simulink model "Comau_endeff_Comp"  (R2024b)
settings: Solver=FixedStepAuto  StartTime=0.0  StopTime=inf  FixedStep=Ts  RelTol=1e-3
model workspace (MATLAB code in the model file):
  other statements: smiDataRobot.RigidTransform(16).translation = [0.0 0.0 0.0];; smiDataRobot.RigidTransform(16).angle = 0.0;; smiDataRobot.RigidTransform(16).axis = [0.0 0.0 0.0];; smiDataRobot.RigidTransform(16).ID = "";; smiDataRobot.RigidTransform(1).translation = [0 331 0];  % mm; smiDataRobot.RigidTransform(1).angle = 0;  % rad; smiDataRobot.RigidTransform(1).axis = [0 0 0];; smiDataRobot.RigidTransform(1).ID = "AssemblyGround[SMART-5 NJ-110-3.0 (3D-STEP).STEP-1:SMART-5 NJ-110-3.0_p02.STEP-1]";; smiDataRobot.RigidTransform(2).translation = [-450 2240 0];  % mm; smiDataRobot.RigidTransform(2).angle = 0;  % rad; smiDataRobot.RigidTransform(2).axis = [0 0 0];; smiDataRobot.RigidTransform(2).ID = "AssemblyGround[SMART-5 NJ-110-3.0 (3D-STEP).STEP-1:SMART-5 NJ-110-3.0_p05.STEP-1]"; ... (+161)
values from neighbouring files (symbols this model uses):
  BList = Adjoint(M_B) * SList    [Comau_robot_3dof_parameters.m]
  M = [1 0 0 L1+L5+L6+L7 ... (first row only)    [Comau_robot_3dof_parameters.m]
  M_B = TransInv(M)    [Comau_robot_3dof_parameters.m]
  SList = [omega_mat; v_mat]    [Comau_robot_3dof_parameters.m]
  thetaList0 = [0 0 0 0 0]    [Comau_robot_3dof_parameters.m]
  tr_p_c = [-1.082024099747949, 1.536041691521612, -0.3]    [Comau_robot_3dof_parameters.m]
  tr_w_p = [-2.969661622702265, 1.976311036084776, 3.312845015592614]    [Comau_robot_3dof_parameters.m]
undefined symbols (not defined in the file or in its folder): L2, L3, L4, SF_x, SF_y, SF_z, smiDataRobot, X, Y, Z
libraries: sm_lib x96, nesl_utility x69, slrealtimeutilitieslib x2, slrealtimeiplib x2, simulink x1, aerolibanimutils x1
(part 5 of 5)

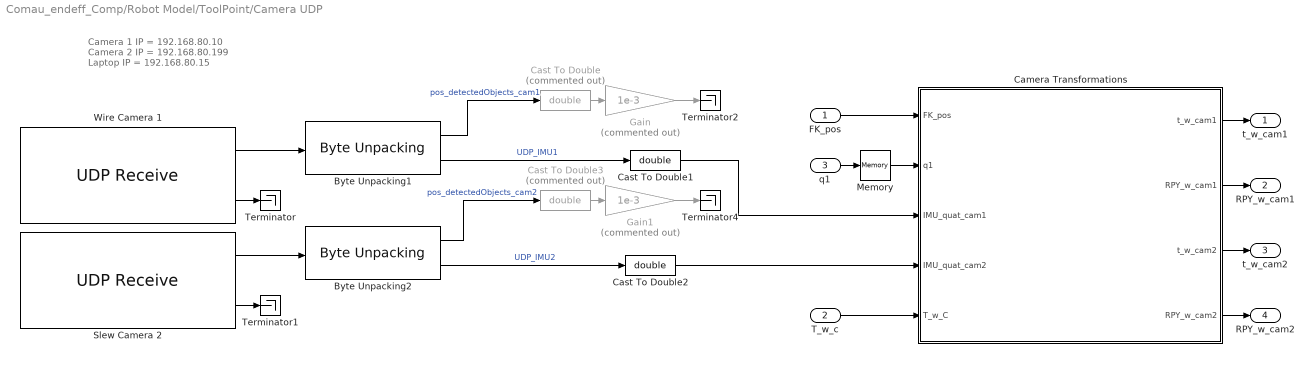
== system Comau_endeff_Comp/Robot Model/ToolPoint/Camera UDP ==
  note: Camera 1 IP = 192.168.80.10
      | Camera 2 IP = 192.168.80.199
      | Laptop IP      = 192.168.80.15
  FK_pos : Inport
  T_w_c : Inport  Port=2
  q1 : Inport  Port=3
  Byte Unpacking1 : slrealtimeutilitieslib/Byte Unpacking  MaskUnpackedDataTypes={'int16', 'single'}  MaskUnpackedDataSizes={[6], [4]}  MaskAlignment=1
  Byte Unpacking2 : slrealtimeutilitieslib/Byte Unpacking  MaskUnpackedDataTypes={'int16', 'single'}  MaskUnpackedDataSizes={[6], [4]}  MaskAlignment=1
  Camera Transformations : MATLAB Function  TreatAsAtomicUnit=on
  Cast To Double : DataTypeConversion  Commented=on  OutDataTypeStr=double  SaturateOnIntegerOverflow=off  RndMeth=Floor
  Cast To Double1 : DataTypeConversion  OutDataTypeStr=double  SaturateOnIntegerOverflow=off  RndMeth=Floor
  Cast To Double2 : DataTypeConversion  OutDataTypeStr=double  SaturateOnIntegerOverflow=off  RndMeth=Floor
  Cast To Double3 : DataTypeConversion  Commented=on  OutDataTypeStr=double  SaturateOnIntegerOverflow=off  RndMeth=Floor
  Gain : Gain  Commented=on  Gain=1e-3
  Gain1 : Gain  Commented=on  Gain=1e-3
  Memory : Memory
  Slew Camera 2 : slrealtimeiplib/UDP Receive  useHostTargetConn=on  ipAddress=192.168.5.80  localPort=5007  rcvWidth=28  rcvFmAny=on  fmAddress='10.10.10.10'  sampleTime=Ts  enableMessage=off  maxPackets=1
  Terminator{,1..2,4} (4 alike) : Terminator
  Wire Camera 1 : slrealtimeiplib/UDP Receive  useHostTargetConn=on  ipAddress=192.168.5.80  localPort=5008  rcvWidth=28  rcvFmAny=on  fmAddress='10.10.10.10'  sampleTime=Ts  enableMessage=off  maxPackets=1
  t_w_cam1 : Outport
  RPY_w_cam1 : Outport  Port=2
  t_w_cam2 : Outport  Port=3
  RPY_w_cam2 : Outport  Port=4
  wires:
  Byte Unpacking1/1 -> Cast To Double/1  "pos_detectedObjects_cam1"
  Wire Camera 1/1 -> Byte Unpacking1/1
  Wire Camera 1/2 -> Terminator/1
  Byte Unpacking1/2 -> Cast To Double1/1  "UDP_IMU1"
  Cast To Double/1 -> Gain/1
  FK_pos/1 -> Camera Transformations/1(FK_pos)
  Camera Transformations/1(t_w_cam1) -> t_w_cam1/1
  Cast To Double1/1 -> Camera Transformations/3(IMU_quat_cam1)
  Camera Transformations/2(RPY_w_cam1) -> RPY_w_cam1/1
  q1/1 -> Memory/1
  Memory/1 -> Camera Transformations/2(q1)
  T_w_c/1 -> Camera Transformations/5(T_w_C)
  Camera Transformations/4(RPY_w_cam2) -> RPY_w_cam2/1
  Camera Transformations/3(t_w_cam2) -> t_w_cam2/1
  Slew Camera 2/2 -> Terminator1/1
  Slew Camera 2/1 -> Byte Unpacking2/1
  Cast To Double2/1 -> Camera Transformations/4(IMU_quat_cam2)
  Byte Unpacking2/2 -> Cast To Double2/1  "UDP_IMU2"
  Byte Unpacking2/1 -> Cast To Double3/1  "pos_detectedObjects_cam2"
  Gain/1 -> Terminator2/1
  Cast To Double3/1 -> Gain1/1
  Gain1/1 -> Terminator4/1

== matlab function Comau_endeff_Comp/TrajectoryGen ==
  settings: updateMethod=DISCRETE
  data: points_x input; points_y input; points_z input; p output size=[1 3]; t input; t_points input; new_command input; traj_method input; p_vel output size=[1 3]; v_max input; traj_running output boolean size=1
function [p, p_vel, traj_running] = TrajectoryGen(points_x, points_y, points_z, t, t_points, new_command, traj_method, v_max)
%#codegen
% TrajectoryGen generates a 3D trajectory based on input waypoints.
%
% Inputs:
%   points_x, points_y, points_z - waypoint vectors or single values
%   depending on trajecotry generator mode (traj_method)
%   t      - current time (scalar)
%   t_points - vector of time stamps for the trajectory
%   new_command - a command counter (as single)
%
% Outputs:
%   p, p_vel - current position and velocity (1x3 vectors)
%   abs_tf_log, base_t_log, local_t, local_tf - diagnostic time variables

% Pre-allocate outputs:
p = zeros(1, 3);
p_vel = zeros(1, 3);

%Traj method for poly spline trajectory
%method = 'quintic';

% Persistent variables for timing and command tracking, and to hold new parameters:
persistent abs_tf base_t last_command 
persistent new_points_x new_points_y new_points_z new_t_points

% Removed cast: t = single(t);

if isempty(abs_tf)
    base_t = 0;
    abs_tf = 0;
end
if isempty(last_command)
    last_command = 0;
end

% Initialize captured parameters if empty:
if isempty(new_points_x)
    new_points_x = points_x;
end
if isempty(new_points_y)
    new_points_y = points_y;
end
if isempty(new_points_z)
    new_points_z = points_z;
end
if isempty(new_t_points)
    new_t_points = t_points;
end

% Detect a new trajectory command:
if new_command ~= last_command
    % Capture the current time as the start:
    base_t = t;
    
    % Capture the new parameters so they remain consistent:
    new_points_x = points_x;
    new_points_y = points_y;
    new_points_z = points_z;
    
    % Calculate the trajectory duration T based on Vmax.
    % Ensure Vmax is not too small and set a minimum time:
    T_min = 1e-6;
    v_max = max(v_max, T_min);
    
    % For a two-point trajectory, use the difference between the first two points.
    T_x = abs(new_points_x(2) - new_points_x(1)) / v_max;
    T_y = abs(new_points_y(2) - new_points_y(1)) / v_max;
    T_z = abs(new_points_z(2) - new_points_z(1)) / v_max;
    
    % Choose the maximum time required among all three axes:
    T = max([T_x, T_y, T_z, T_min]);
    
    % Set the absolute finish time based on the computed duration:
    abs_tf = T + t;
    
    % (Optionally) store T in new_t_points if needed
    new_t_points = T;  
    
    % Update the command counter:
    last_command = new_command;
end

% Compute local time variables:
local_t = t - base_t;
local_tf = abs_tf - base_t;


%maybe not need keep for now
% Clamp local_t so it doesn't exceed the final time:
%if traj_method ~= 3
%    if local_t > local_tf
%        local_t = local_tf;
%    end
%end

% Compute the trajectory:
if abs_tf == 0 || v_max == 0 % Stay in current position if Trajectory not initialized OR v_max input = 0
    x_pos = new_points_x(1);
    y_pos = new_points_y(1);
    z_pos = new_points_z(1);
    
    x_vel = 0;
    y_vel = 0;
    z_vel = 0;
else
    if traj_method == 1
        [x_pos, x_vel, ~] = cubicTrajectoryPlanner(local_t, local_tf, new_points_x(1), new_points_x(2), 0, 0);
        [y_pos, y_vel, ~] = cubicTrajectoryPlanner(local_t, local_tf, new_points_y(1), new_points_y(2), 0, 0);
        [z_pos, z_vel, ~] = cubicTrajectoryPlanner(local_t, local_tf, new_points_z(1), new_points_z(2), 0, 0);
        
        %VMax
        %[x_pos, x_vel, ~] = cubicTrajectoryPlanner_Vmax(local_t, v_max, new_points_x(1), new_points_x(2), 0, 0);
        %[y_pos, y_vel, ~] = cubicTrajectoryPlanner_Vmax(local_t, v_max, new_points_y(1), new_points_y(2), 0, 0);
        %[z_pos, z_vel, ~] = cubicTrajectoryPlanner_Vmax(local_t, v_max, new_points_z(1), new_points_z(2), 0, 0);
    elseif traj_method == 2
        %Quintic [pos, vel, acc] = quinticTrajectoryPlanner(t, T, P0, Pf, V0, Vf, A0, Af)
        [x_pos, x_vel, ~] = quinticTrajectoryPlanner(local_t, local_tf, new_points_x(1), new_points_x(2), 0, 0, 0, 0);
        [y_pos, y_vel, ~] = quinticTrajectoryPlanner(local_t, local_tf, new_points_y(1), new_points_y(2), 0, 0, 0, 0);
        [z_pos, z_vel, ~] = quinticTrajectoryPlanner(local_t, local_tf, new_points_z(1), new_points_z(2), 0, 0, 0, 0);
        
        %VMax
        %[x_pos, x_vel, ~] = quinticTrajectoryPlanner_Vmax(local_t, v_max, new_points_x(1), new_points_x(2), 0, 0, 0, 0);
        %[y_pos, y_vel, ~] = quinticTrajectoryPlanner_Vmax(local_t, v_max, new_points_y(1), new_points_y(2), 0, 0, 0, 0);
        %[z_pos, z_vel, ~] = quinticTrajectoryPlanner_Vmax(local_t, v_max, new_points_z(1), new_points_z(2), 0, 0, 0, 0);
    elseif traj_method == 3
        method = 'quintic';
        %Multi point online trajectory planner here
        %[x_pos, x_vel, ~, ~] = multipointTrajectorySplineAuto(local_t, new_points_x, v_max, method);
        %[y_pos, y_vel, ~, ~] = multipointTrajectorySplineAuto(local_t, new_points_y, v_max, method);
        %[z_pos, z_vel, ~, ~] = multipointTrajectorySplineAuto(local_t, new_points_z, v_max, method);

        x_pos = new_points_x(1);
        y_pos = new_points_y(1);
        z_pos = new_points_z(1);
        
        x_vel = 0;
        y_vel = 0;
        z_vel = 0;
    else %Defualt cubic
        [x_pos, x_vel, ~] = cubicTrajectoryPlanner(local_t, local_tf, new_points_x(1), new_points_x(2), 0, 0);
        [y_pos, y_vel, ~] = cubicTrajectoryPlanner(local_t, local_tf, new_points_y(1), new_points_y(2), 0, 0);
        [z_pos, z_vel, ~] = cubicTrajectoryPlanner(local_t, local_tf, new_points_z(1), new_points_z(2), 0, 0);
    end
end


p(1) = x_pos;
p(2) = y_pos;
p(3) = z_pos;

p_vel(1) = x_vel;
p_vel(2) = y_vel;
p_vel(3) = z_vel;

traj_running = (t <= abs_tf + 0.1); %Trajectory complete flag with 0.1 second buffer

traj_running = logical(traj_running);
end

== matlab function Comau_endeff_Comp/Robot Model/ToolPoint/Camera UDP/Camera Transformations ==
  data: t_w_cam1 output; FK_pos input; q1 input; IMU_quat_cam1 input; IMU_quat_cam2 input; RPY_w_cam1 output; t_w_cam2 output; T_w_C input; RPY_w_cam2 output
function [t_w_cam1, RPY_w_cam1, t_w_cam2, RPY_w_cam2] = transformFrame(FK_pos, q1, IMU_quat_cam1, IMU_quat_cam2, T_w_C)

    % FK_pos = t_w_ee
% World to End Effector
R_w_ee = rotz_deg(-q1);
% t_C_ee_homog = [FK_pos; 1];
% t_w_ee_homog = T_w_C * t_C_ee_homog;
% t_w_ee = t_w_ee_homog(1:3);
t_w_ee = FK_pos + T_w_C(1:3, 4);
T_w_ee = [R_w_ee, t_w_ee; 
           0 0 0,      1 ];

%%% Common for all OAK D Pro Cameras %%%
% Camera frame to IMU
R_cam_IMU = roty_deg(-90);
t_cam_IMU = [-1.18 ; 4.50 ; -27.25 ]*1e-3; % [m]
T_cam_IMU = [R_cam_IMU , t_cam_IMU;
                 0 0 0 ,         1 ];

% % Camera frame to RGB
% R_cam_RGB = 0; % <<<<<<<<<<<<<<<<<<<<<<<<<<<<<<<<<<<<<<<
% t_cam_RGB = [ 7.2 ; 44.5 ; -6.9867 ]*1e-3; % [m]
% T_cam_RGB = [ R_cam_RGB , t_cam_RGB;
%                   0 0 0 ,         1 ];
%%% Common for all OAK D Pro Cameras %%%

%% Wire Camera

% Reorder quaternion from [x; y; z; w] to MATLAB's expected [w, x, y, z]
q1 = [IMU_quat_cam1(4), IMU_quat_cam1(1), IMU_quat_cam1(2), IMU_quat_cam1(3)];
% Convert quaternion to rotation matrix (using MATLAB's Aerospace Toolbox convention)
% Cam_RPY1 = quat2eul(q1);
% Cam_RPY1 = rad2deg(Cam_RPY1);
R_IMU1 = quat2rotm(q1);
R_cam1 = R_IMU1 * R_cam_IMU'; % Transpose to reverse

% Known translation (offset) from the end effector (EE) to camera 1
t_ee_cam1 = [-0.10; 0; -0.50];
% Combine the IMU rotation with the fixed offset
T_ee_cam1 = [R_cam1, t_ee_cam1; 0 0 0 1];
% World to camera
T_w_cam1 = T_w_ee * T_ee_cam1;

% Extract translation & orientation from transformation matrix
t_w_cam1 = T_w_cam1(1:3,4);
R_w_cam1 = T_w_cam1(1:3,1:3);
RPY_w_cam1 = rotm2eul(R_w_cam1, 'XYZ');
t_w_cam1 = T_w_ee(1:3, 4);

% % Unused? - TLS
% R_offset = roty_deg(-pi) * rotz_deg(-pi/2);
% T_offset = [R_offset, zeros(3,1); 0 0 0 1];

%% Slew Camera
    % p0X are component names in SolidWorks files

% % From COMAU to p01
% R_C_p01 = rotx_deg(-90)*rotz_deg(180);
% T_C_p01 = [R_C_p01, [0;0;0];
%              0 0 0,       1 ];

% From p01 to p02
t_p01_p02 = [0; 126; 0]*1e-3; % [m]
R_p01_p02 = eye(3);
T_p01_p02 = [R_p01_p02, t_p01_p02;
                 0 0 0,         1 ];

% From p02 to camera 2
R_p02_cam2 = roty_deg(20);
t_p02_cam2 = [ 572.11 ; -43.50 ; 106.55 ]*1e-3; % [m]
T_p02_cam2 = [R_p02_cam2, t_p02_cam2;
                 0 0 0,         1 ];

% From p01 to camera 2
T_p01_cam2 = T_p01_p02 * T_p02_cam2;

% From World to camera 2
T_w_cam2 = T_w_C * T_p01_cam2; % p01 = COMAU frame

% Reorder quaternion from [x; y; z; w] to MATLAB's expected [w, x, y, z]
q2 = [IMU_quat_cam2(4), IMU_quat_cam2(1), IMU_quat_cam2(2), IMU_quat_cam2(3)];
R_w_IMU2 = quat2rotm(q2);
R_w_cam2 = R_w_IMU2 * R_cam_IMU'; % Transpose to reverse
% RPY_w_cam2 = quat2eul(q2);

% Extract translation & orientation from transformation matrix
t_w_cam2 = T_w_cam2(1:3, 4);
% R_w_cam2 = T_w_cam2(1:3, 1:3);
RPY_w_cam2 = rotm2eul(R_w_cam2, 'XYZ');


end

%% 
function R = rotx_deg(theta)
    R = [ 1           0            0;
          0 cosd(theta) -sind(theta);
          0 sind(theta)  cosd(theta) ];
end

function R = roty_deg(theta)
    R = [ cosd(theta)  0 sind(theta);
          0            1           0;
         -sind(theta)  0 cosd(theta) ];
end

function R = rotz_deg(theta)
    R = [cosd(theta) -sind(theta) 0;
         sind(theta)  cosd(theta) 0;
                   0            0 1];
end

== stateflow chart Comau_endeff_Comp/Chart ==
  state Go_home
    entry:
    X_home = 2.62;
    Y_home = 0;
    Z_home = 2.24;
    Traj_points_XYZ = [FK_Pos(1), X_home, FK_Pos(2), Y_home, FK_Pos(3), Z_home];
    Traj_method = 2;
    v_max = 0.1;
    new_command = new_command + 1;
  state Stay_in_current_position
    entry:
    % Set the values for the variables
    Traj_points_XYZ = [FK_Pos(1), FK_Pos(1), FK_Pos(2), FK_Pos(2), FK_Pos(3), FK_Pos(3)];
    Traj_method = 1;
    v_max = 0;
    new_command = new_command + 1;
  state Move_to_above_platform
    %Move above platform to initiate hooking procedure
    %Revieve in testing later if this stage is necessery or can be optimized
    entry:
    X_Platform = 3.14;
    Y_Platform = 0.4;
    Z_Platform = 2.0;
    Traj_points_XYZ = [FK_Pos(1), X_Platform, FK_Pos(2), Y_Platform, FK_Pos(3), Z_Platform];
    Traj_method = 2;
    v_max = 0.1;
    new_command = new_command + 1;
  state Hook_Ball
    state Move_Close_To_Ball
      entry:
      X_Offset = -0.24;
      Y_Offset = -0.24;
      Z_Offset = -0.07;
      Target_Pos_X = Ball_Pos(1) + X_Offset;
      Target_Pos_Y = Ball_Pos(2) + Y_Offset;
      Target_Pos_Z = Ball_Pos(3) +  Winch_length; %Z_Offset + Claw_Pos(3);
      Traj_points_XYZ = [FK_Pos(1), Target_Pos_X, FK_Pos(2), Target_Pos_Y, FK_Pos(3), Target_Pos_Z];
      Traj_method = 2;
      v_max = 0.1;
      new_command = new_command + 1;
      during:
      if ~traj_running
      Sub_stage_switch = 2;
      else
      Sub_stage_switch = 1;
      end
    state Ball_In_Frame
      if all(abs(Ball_Pos) < 20)
      Sub_stage_switch = 1;
      else
      Sub_stage_switch = 0;
      v_max = 0;
      end
    state Move_in_to_ball
      entry:
      Traj_points_XYZ = [FK_Pos(1), Ball_Pos(1), FK_Pos(2), Ball_Pos(2), FK_Pos(3), Ball_Pos(3)+Winch_length ];
      Traj_method = 2;
      v_max = 0.02;
      new_command = new_command + 1;
      during:
      if ~traj_running
      Sub_stage_switch = 3;
      else
      Sub_stage_switch = 2;
      end
    state Lift_Up
      entry:
      Z_Up = FK_Pos(3) + 0.20;
      Traj_points_XYZ = [FK_Pos(1), FK_Pos(1), FK_Pos(2), FK_Pos(2), FK_Pos(3), Z_Up ];
      Traj_method = 2;
      v_max = 0.05;
      new_command = new_command + 1;
    (default) -> Ball_In_Frame
    Ball_In_Frame -> Move_Close_To_Ball : [Sub_stage_switch == 1]
    Move_Close_To_Ball -> Move_in_to_ball : [Sub_stage_switch == 2]
    Move_in_to_ball -> Lift_Up : [Sub_stage_switch == 3]
  (default) -> Stay_in_current_position
  Hook_Ball -> Go_home [order 3] : [Switch == 1]
  Stay_in_current_position -> Go_home [order 1] : [Switch == 1]
  Go_home -> Stay_in_current_position [order 1] : [Switch == 0]
  Hook_Ball -> Stay_in_current_position [order 2] : [Switch == 0]
  Move_to_above_platform -> Stay_in_current_position [order 1] : [Switch == 0]
  Stay_in_current_position -> Move_to_above_platform [order 2] : [Switch == 2]
  Move_to_above_platform -> Go_home [order 2] : [Switch == 1]
  Go_home -> Move_to_above_platform [order 2] : [Switch == 2]
  Move_to_above_platform -> Hook_Ball [order 3] : [Switch == 3]
  Hook_Ball -> Move_to_above_platform [order 1] : [Switch==2]
  data: Switch input; Traj_points_XYZ output; new_command output =0; Traj_method output; v_max output =0; FK_Pos input; Claw_Pos input; Z_home local; X_home local; Y_home local; X_Platform local; Z_Platform local; Y_Platform local; Ball_Pos input; Winch_length input; Z_Offset local; X_Offset local; Target_Pos_Y local; Target_Pos_X local; Target_Pos_Z local; Y_Offset local; Sub_stage_switch local; traj_running input; Z_Up local

== matlab function Comau_endeff_Comp/MATLAB Function1 ==
  data: Em8000_RPY input; R output
function R = RotMat(Em8000_RPY)

% Convert from Euler Angle to Rodrigues Vector
R = eul2rotm( [Em8000_RPY(1) Em8000_RPY(2) Em8000_RPY(3)] , 'XYZ');

== matlab function Comau_endeff_Comp/Robot Model/ToolPoint/MATLAB Function ==
  data: T_w_C input; t_w_C output; RPY_w_C output
function [ t_w_C , RPY_w_C ] = fcn(T_w_C)

t_w_C = T_w_C(1:3, 4);
R_w_C = T_w_C(1:3, 1:3);
RPY_w_C = rotm2eul(R_w_C, 'XYZ');

== matlab function Comau_endeff_Comp/Forward Kinematics ==
  data: thetalist input; t_C_ee output; T_w_C output; M input; SList input; T_C_ee output; t_w_ee output; Em8000_RPY input; Em8000_tr input
function [t_C_ee, T_w_C, T_C_ee, t_w_ee]  = FK_cartPos(thetalist, M, SList, Em8000_RPY, Em8000_tr)
% Compute end effector frame from Forward kinematics to measure end effector position
T_C_ee = FKinSpace(M,SList,thetalist); % Keep in local robot base frame coordinates for IK solver

t_C_ee = [T_C_ee(1:3,4)];

%% Transform to world frame for trajectory planner 

% World frame to platform frame - From GitLab calibration
w_s_quat = [6.0198987883e-05, 0.705931944115, 0.708279565403954, 0.000379322138596];
R_w_p = quat2rotm(w_s_quat);
tr_w_p = [-2.969661622702265, 1.976311036084776, 2.662845015592614]';
T_w_pStatic = [R_w_p, tr_w_p; zeros(1,3), 1]; % Static transform 

% Platform frame to COMAU - From GitLab calibration
p_C_quat = [0.002461288106714, -0.501408337431486, -0.865206982556575, 0.000706081011787];
R_p_C = quat2rotm(p_C_quat); % rotation matrix
tr_p_C = [-1.082024099747949, 1.536041691521612, -1.024461448780775]'; % Translational vector
T_p_C = [R_p_C, tr_p_C; zeros(1,3), 1]; % Static transformation between platform frame and comau robot base frame

Em8000_RPY = [Em8000_RPY(1) Em8000_RPY(2) Em8000_RPY(3)];
R_pStatic_p = eul2rotm(Em8000_RPY,"XYZ"); % Dynamic rotation of the platform body 

% Transformation matrix of the dynamic movement of the platform (rotation and translation seen from the origin of the platform ie not in world frame)
T_pStatic_p = [R_pStatic_p, Em8000_tr; zeros(1,3), 1];

% World frame to moving platform frame
T_w_p = T_w_pStatic * T_pStatic_p;

% World frame to COMAU
T_w_C = T_w_p * T_p_C;

% World frame to End Effector
T_w_ee = T_w_C * T_C_ee;

t_w_ee = [T_w_ee(1:3,4)];

== matlab function Comau_endeff_Comp/inverseKinematics ==
  data: thetaListDot output; Em8000_tr input; Em8000_vel input; unused input; Em8000_RPY input; T_C_ee input; Traj_vel input; thetaList0 input; BList input; R_dot input; R input
function thetaListDot  = inverseKinematics( ...
    Em8000_tr,  Em8000_vel, ~, Em8000_RPY, T_C_ee, Traj_vel, thetaList0, BList,R_dot,R)

%% From FK

% World frame to platform frame - From GitLab calibration
w_s_quat = [6.0198987883e-05, 0.705931944115, 0.708279565403954, 0.000379322138596];
R_w_p = quat2rotm(w_s_quat);
tr_w_p = [-2.969661622702265, 1.976311036084776, 2.662845015592614]';
T_w_pStatic = [R_w_p, tr_w_p; zeros(1,3), 1]; % Static transform 

% Platform frame to COMAU - From GitLab calibration
p_C_quat = [0.002461288106714, -0.501408337431486, -0.865206982556575, 0.000706081011787];
R_p_C = quat2rotm(p_C_quat); % rotation matrix
tr_p_C = [-1.082024099747949, 1.536041691521612, -1.024461448780775]'; % Translational vector
T_p_C = [R_p_C, tr_p_C; zeros(1,3), 1]; % Static transformation between platform frame and comau robot base frame

Em8000_RPY = [Em8000_RPY(1) Em8000_RPY(2) Em8000_RPY(3)];
R_pStatic_pDynamic = eul2rotm(Em8000_RPY,"XYZ"); % Dynamic rotation of the platform body 

% Transformation matrix of the dynamic movement of the platform (rotation and translation seen from the origin of the platform ie not in world frame)
T_pStatic_pDynamic = [R_pStatic_pDynamic, Em8000_tr; zeros(1,3), 1];

% World frame to moving platform frame
T_w_p = T_w_pStatic * T_pStatic_pDynamic;

% World frame to COMAU
T_w_C = T_w_p * T_p_C;

% World frame to End Effector
T_w_ee = T_w_C * T_C_ee;
    % t_w_ee = [T_w_ee(1:3,4)];

%% Specific for Inverse Kinematics
Jb = JacobianBody(BList,thetaList0);

Jb_pinv = pinv(Jb);

% Desired end effector twist vector of trajectory
V_w_traj =  [0;
         0;
         0;
         Traj_vel(1);
         Traj_vel(2);
         Traj_vel(3)
         ];

Omega = R_dot*R'; % Skew Symmetric Matrix
Em8000_omega = [Omega(3,2) ; Omega(1,3) ; Omega(2,1) ]; % Extract Angular Velocity Vector

% Twist vector of platform motion
V_p =   [Em8000_omega(1);
         Em8000_omega(2);
         Em8000_omega(3);
         Em8000_vel(1);
         Em8000_vel(2);
         Em8000_vel(3)
         ];

% Twist vector of platform expressed in world frame
V_w_p = Adjoint(T_w_p) * V_p;

% Twist vector of platform expressed in dynamic robot end effector frame
V_ee_p = Adjoint(TransInv(T_w_ee)) * V_w_p;
% Twist vector of trajectory expressed in dynamic robot end effector frame
V_ee_traj = Adjoint(TransInv(T_w_ee)) * V_w_traj;

% Inverse velocity kinematics mr chapter 6.3
thetaListDot = Jb_pinv * (V_ee_traj - V_ee_p);

end
